simulink model "kuka_admittance"  (R2019b)
settings: Solver=ode1  StartTime=0.0  StopTime=t(end)  FixedStep=dt  RelTol=1e-3
model workspace (MAT data in the model file):
  SL_ROS_VariableLengthArrays_MaxSizes.CommonInfo.ArrayTruncateAction = 'EmitWarning'
  SL_ROS_VariableLengthArrays_MaxSizes.MsgTypeMap = containers.Map
  SL_ROS_VariableLengthArrays_MaxSizes.MsgTypeMap.serialization.keys = {'iiwa_py4j_pkg/ExternalTorque', 'iiwa_py4j_pkg/JointCommandPosition', 'ros_iiwa_fri/ExternalTorque', 'ros_iiwa_fri/JointCommandPosition', 'sensor_msgs/JointState'}
  SL_ROS_VariableLengthArrays_MaxSizes.MsgTypeMap.serialization.values{1}.PropertyName = 'Values'
  SL_ROS_VariableLengthArrays_MaxSizes.MsgTypeMap.serialization.values{1}.DataType = 'single'
  SL_ROS_VariableLengthArrays_MaxSizes.MsgTypeMap.serialization.values{1}.MaxLength = 7
  SL_ROS_VariableLengthArrays_MaxSizes.MsgTypeMap.serialization.values{2}.PropertyName = 'Values'
  SL_ROS_VariableLengthArrays_MaxSizes.MsgTypeMap.serialization.values{2}.DataType = 'single'
  SL_ROS_VariableLengthArrays_MaxSizes.MsgTypeMap.serialization.values{2}.MaxLength = 7
  SL_ROS_VariableLengthArrays_MaxSizes.MsgTypeMap.serialization.values{3}.PropertyName = 'Values'
  SL_ROS_VariableLengthArrays_MaxSizes.MsgTypeMap.serialization.values{3}.DataType = 'double'
  SL_ROS_VariableLengthArrays_MaxSizes.MsgTypeMap.serialization.values{3}.MaxLength = 7
  SL_ROS_VariableLengthArrays_MaxSizes.MsgTypeMap.serialization.values{4}.PropertyName = 'Values'
  SL_ROS_VariableLengthArrays_MaxSizes.MsgTypeMap.serialization.values{4}.DataType = 'double'
  SL_ROS_VariableLengthArrays_MaxSizes.MsgTypeMap.serialization.values{4}.MaxLength = 7
  SL_ROS_VariableLengthArrays_MaxSizes.MsgTypeMap.serialization.values{5}(1).PropertyName = 'Effort'
  SL_ROS_VariableLengthArrays_MaxSizes.MsgTypeMap.serialization.values{5}(1).DataType = 'double'
  SL_ROS_VariableLengthArrays_MaxSizes.MsgTypeMap.serialization.values{5}(1).MaxLength = 128
  SL_ROS_VariableLengthArrays_MaxSizes.MsgTypeMap.serialization.values{5}(2).PropertyName = 'Name'
  SL_ROS_VariableLengthArrays_MaxSizes.MsgTypeMap.serialization.values{5}(2).DataType = 'std_msgs/String'
  SL_ROS_VariableLengthArrays_MaxSizes.MsgTypeMap.serialization.values{5}(2).MaxLength = 16
  SL_ROS_VariableLengthArrays_MaxSizes.MsgTypeMap.serialization.values{5}(3).PropertyName = 'Position'
  SL_ROS_VariableLengthArrays_MaxSizes.MsgTypeMap.serialization.values{5}(3).DataType = 'double'
  SL_ROS_VariableLengthArrays_MaxSizes.MsgTypeMap.serialization.values{5}(3).MaxLength = 7
  SL_ROS_VariableLengthArrays_MaxSizes.MsgTypeMap.serialization.values{5}(4).PropertyName = 'Velocity'
  SL_ROS_VariableLengthArrays_MaxSizes.MsgTypeMap.serialization.values{5}(4).DataType = 'double'
  SL_ROS_VariableLengthArrays_MaxSizes.MsgTypeMap.serialization.values{5}(4).MaxLength = 128
  SL_ROS_VariableLengthArrays_MaxSizes.MsgTypeMap.serialization.uniformity = 0
  SL_ROS_VariableLengthArrays_MaxSizes.MsgTypeMap.serialization.keyType = 'char'
  SL_ROS_VariableLengthArrays_MaxSizes.MsgTypeMap.serialization.valueType = 'any'
values from neighbouring files (symbols this model uses):
  dt = 0.002    [run_this_first.m]
  q_0 = mean_motion.signals.values(1,:)    [run_this_first.m]
undefined symbols (not defined in the file or in its folder): Stamp, Values, Values_SL_Info
libraries: robotlib x5
settings Model: EnablePacing=on  Creator=mojo  LastModifiedBy=johannesmogster
settings OptimizationCC: EnhancedBackFolding=on  PassReuseOutputArgsAs=Individual arguments  ZeroExternalMemoryAtStartup=off  ZeroInternalMemoryAtStartup=off  MaxStackSize=64  OptimizeBlockOrder=speed  DifferentSizesBufferReuse=on  OptimizationCustomize=off  EfficientTunableParamExpr=on
settings DebuggingCC: ParameterTunabilityLossMsg=error
settings HardwareCC: ProdBitPerPointer=32  ProdBitPerSizeT=32  ProdBitPerPtrDiffT=32  ProdLargestAtomicFloat=None  ProdIntDivRoundTo=Undefined  ProdEndianess=Unspecified  ProdWordSize=32  ProdHWDeviceType=Generic->Unspecified (assume 32-bit Generic)
settings SFSimCC: MATLABDynamicMemAlloc=off
settings RTWCC: SystemTargetFile=ert.tlc  HardwareBoard=Robot Operating System (ROS)  TLCOptions="-aInlineSetEventsForThisBaseRateFcn=TLC_FALSE -aSuppressMultiTaskScheduler=TLC_FALSE  -aRateBasedStepFcn=0"  TemplateMakefile=ert_default_tmf  GenerateReport=on  Toolchain=Catkin  IncludeHyperlinkInReport=on  LaunchReport=on  TargetLang=C++  GenerateTraceInfo=on  GenerateTraceReport=on  GenerateTraceReportSl=on  GenerateTraceReportSf=on  GenerateTraceReportEml=on
settings CodeAppCC: ForceParamTrailComments=on  IgnoreCustomStorageClasses=off  OperatorAnnotations=on  SimulinkDataObjDesc=on  SFDataObjDesc=on  InsertBlockDesc=on
settings ERTTargetCC: SupportContinuousTime=on  SupportVariableSizeSignals=on

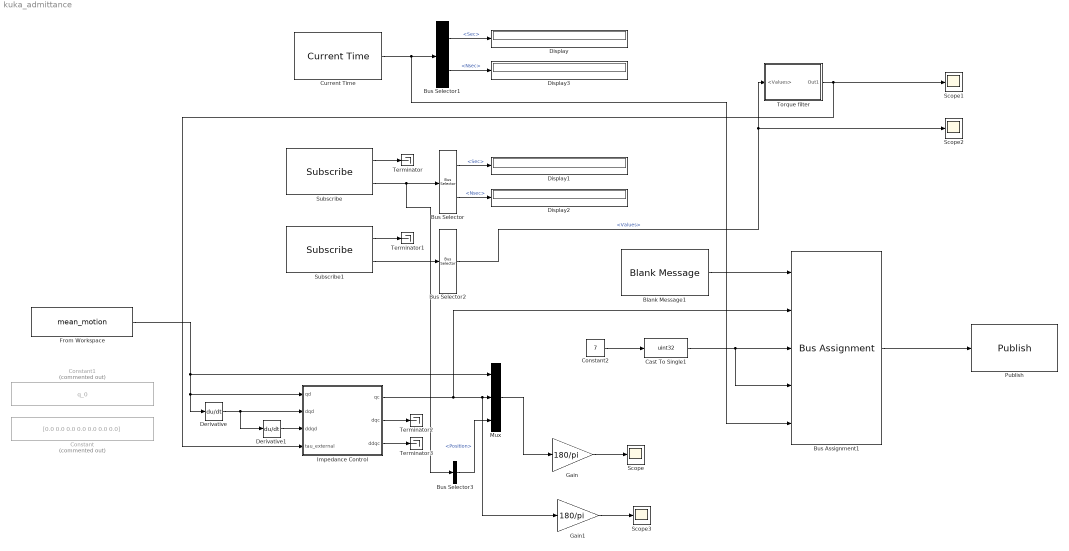
== system kuka_admittance ==
  Blank Message1 : robotlib/Blank Message  messageClass=Message  entityType=ros_iiwa_fri/JointCommandPosition  messageType=ros_iiwa_fri/JointCommandPosition  SampleTime=inf
      settings: SourceProductName=ROS Toolbox
  Bus Assignment1 : BusAssignment  AssignedSignals=Values,Values_SL_Info.CurrentLength,Values_SL_Info.ReceivedLength,Stamp
  Bus Selector : BusSelector  OutputSignals=Header.Stamp.Sec,Header.Stamp.Nsec
  Bus Selector1 : BusSelector  OutputSignals=Sec,Nsec
  Bus Selector2 : BusSelector  OutputSignals=Values
  Bus Selector3 : BusSelector  OutputSignals=Position
  Cast To Single1 : DataTypeConversion  OutDataTypeStr=uint32
  Constant : Constant  Commented=on  Value=[0.0 0.0 0.0 0.0 0.0 0.0 0.0]
  Constant1 : Constant  Commented=on  Value=q_0  SampleTime=dt
  Constant2 : Constant  Value=7
  Current Time : robotlib/Current Time  OutputFormat=bus  SampleTime=-1  ModelName=kuka_admittance
      settings: SourceProductName=ROS Toolbox  SourceProductBaseCode=RR
  Derivative : Derivative
  Derivative1 : Derivative
  Display{,1..3} (4 alike) : Display
  From Workspace : FromWorkspace  VariableName=mean_motion  SampleTime=dt  OutputAfterFinalValue=Holding final value
  Gain : Gain  Gain=180/pi
  Gain1 : Gain  Gain=180/pi
  Impedance Control : Subsystem  mask{Kp=[210 210 90 60 20 15 2], damping_ratio=[0.9 0.9 0.9 0.7 0.7 0.5 0.7], qc_0=q_0, Md=[40 40 20 10 10 1 0.1]}
      mask prompts: Kp "Kp [Nm/rad]"; damping_ratio "Damping ratio []"
  Mux : Mux  Inputs=3
  Publish : robotlib/Publish  topicSource=Select from ROS network  topic=/iiwa_joint_cmd_pos  messageType=ros_iiwa_fri/JointCommandPosition  messageQueueLength=1
      settings: SourceProductName=ROS Toolbox
  Scope{,1..3} (4 alike) : Scope
  Subscribe : robotlib/Subscribe  topicSource=Select from ROS network  topic=/iiwa_joint_states  messageType=sensor_msgs/JointState  sampleTime=-1  messageQueueLength=1
      settings: SourceProductName=ROS Toolbox
  Subscribe1 : robotlib/Subscribe  topicSource=Select from ROS network  topic=/iiwa_external_torque  messageType=ros_iiwa_fri/ExternalTorque  sampleTime=-1  messageQueueLength=1
      settings: SourceProductName=ROS Toolbox
  Terminator{,1..3} (4 alike) : Terminator
  Torque filter : Subsystem
  wires:
  Current Time/1 -> Bus Assignment1/5, Bus Selector1/1
  Bus Selector/1 -> Display1/1  "<Sec>"
  Bus Selector/2 -> Display2/1  "<Nsec>"
  Bus Selector1/1 -> Display/1  "<Sec>"
  Bus Selector1/2 -> Display3/1  "<Nsec>"
  Subscribe/1 -> Terminator/1
  Bus Assignment1/1 -> Publish/1
  Blank Message1/1 -> Bus Assignment1/1
  Constant2/1 -> Cast To Single1/1
  Cast To Single1/1 -> Bus Assignment1/4, Bus Assignment1/3
  Impedance Control/1(qc) -> Bus Assignment1/2, Gain1/1, Mux/2
  Mux/1 -> Gain/1
  Subscribe1/1 -> Terminator1/1
  Subscribe1/2 -> Bus Selector2/1
  Bus Selector2/1 -> Scope2/1, Torque filter/1(<Values>)  "<Values>"
  Derivative/1 -> Derivative1/1, Impedance Control/2(dqd)
  Gain/1 -> Scope/1
  Impedance Control/2(dqc) -> Terminator2/1
  Impedance Control/3(ddqc) -> Terminator3/1
  From Workspace/1 -> Mux/1, Impedance Control/1(qd), Derivative/1
  Torque filter/1(Out1) -> Scope1/1, Impedance Control/4(tau_external)
  Subscribe/2 -> Bus Selector3/1, Bus Selector/1
  Bus Selector3/1 -> Mux/3  "<Position>"
  Gain1/1 -> Scope3/1
  Derivative1/1 -> Impedance Control/3(ddqd)

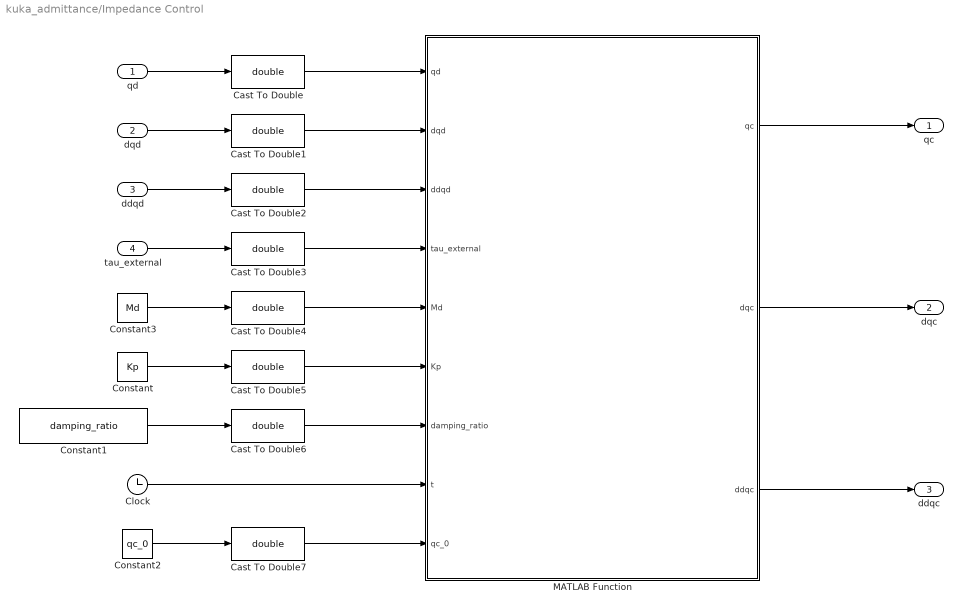
== system kuka_admittance/Impedance Control ==
  qd : Inport
  dqd : Inport  Port=2
  ddqd : Inport  Port=3
  tau_external : Inport  Port=4
  Cast To Double{,1..7} (8 alike) : DataTypeConversion  OutDataTypeStr=double
  Clock : Clock
  Constant : Constant  Value=Kp
  Constant1 : Constant  Value=damping_ratio
  Constant2 : Constant  Value=qc_0
  Constant3 : Constant  Value=Md
  MATLAB Function : MATLAB Function  TreatAsAtomicUnit=on
  qc : Outport
  dqc : Outport  Port=2
  ddqc : Outport  Port=3
  wires:
  tau_external/1 -> Cast To Double3/1
  dqd/1 -> Cast To Double1/1
  ddqd/1 -> Cast To Double2/1
  MATLAB Function/1(qc) -> qc/1
  MATLAB Function/2(dqc) -> dqc/1
  MATLAB Function/3(ddqc) -> ddqc/1
  Constant/1 -> Cast To Double5/1
  Constant1/1 -> Cast To Double6/1
  Clock/1 -> MATLAB Function/8(t)
  Constant2/1 -> Cast To Double7/1
  qd/1 -> Cast To Double/1
  Constant3/1 -> Cast To Double4/1
  Cast To Double/1 -> MATLAB Function/1(qd)
  Cast To Double1/1 -> MATLAB Function/2(dqd)
  Cast To Double2/1 -> MATLAB Function/3(ddqd)
  Cast To Double3/1 -> MATLAB Function/4(tau_external)
  Cast To Double4/1 -> MATLAB Function/5(Md)
  Cast To Double5/1 -> MATLAB Function/6(Kp)
  Cast To Double6/1 -> MATLAB Function/7(damping_ratio)
  Cast To Double7/1 -> MATLAB Function/9(qc_0)

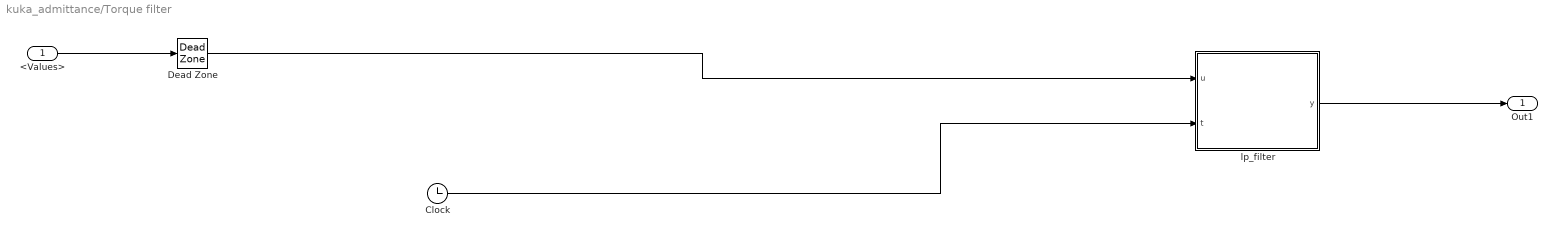
== system kuka_admittance/Torque filter ==
  <Values> : Inport
  Clock : Clock
  Dead Zone : DeadZone  LowerValue=-1  UpperValue=1  SaturateOnIntegerOverflow=on
  lp_filter : MATLAB Function  TreatAsAtomicUnit=on
  Out1 : Outport
  wires:
  lp_filter/1(y) -> Out1/1
  Clock/1 -> lp_filter/2(t)
  <Values>/1 -> Dead Zone/1
  Dead Zone/1 -> lp_filter/1(u)

== matlab function kuka_admittance/Impedance Control/MATLAB Function ==
  settings: updateMethod=DISCRETE
  data: qd input; dqd input; ddqd input; qc output; tau_external input; Md input; Kp input; damping_ratio input; t input; dqc output; ddqc output; qc_0 input
function [qc,dqc, ddqc] = admittance_control(qd,dqd,ddqd,tau_external, ...
    Md, Kp,damping_ratio, ...
    t, qc_0)

Kd = 2*damping_ratio.*sqrt(Md.*Kp);

persistent dqc_prev qc_prev ddqc_prev t_prev
if isempty(dqc_prev)
    dqc_prev = dqd;
    qc_prev = qc_0;
    ddqc_prev = ddqd;
    t_prev = t;
    delta_t = 0.002;
else
    delta_t = t-t_prev;
end


%% Integrate

dqc = dqc_prev + delta_t*ddqc_prev;
qc = qc_prev + delta_t*dqc;

%% Tilde
qc_tilde = qd-qc;
dqc_tilde = dqd-dqc;
ddqc_tilde = Md.^-1.*(-tau_external - Kp.*qc_tilde - Kd.*dqc_tilde);

%%
ddqc = -(ddqc_tilde-ddqd);

%% update storage
ddqc_prev = ddqc;
dqc_prev = dqc;
qc_prev = qc;
t_prev = t;

== matlab function kuka_admittance/Torque filter/lp_filter ==
  settings: updateMethod=DISCRETE
  data: u input; y output; t input
function y  = lp_filter(u,t)
%% Low Pass Filter
% set the time constant, filter out changes faster than that

%% User input
tau = 0.025;

%%

persistent y_prev t_prev
if isempty(y_prev)
    y_prev = u;
    t_prev = t;
    delta_t = 0.002;
else
    delta_t = t-t_prev;
end

a = delta_t/(tau + delta_t);

y = a.*u + (1-a).*y_prev;


%% Memory
t_prev = t;
y_prev = y;
